simulink model "aero_pendulum_state_space"  (R2014a)
settings: Solver=ode45  StartTime=0.0  StopTime=Tsym  MaxStep=Ts  RelTol=1e-3
values from neighbouring files (symbols this model uses):
  A = [0 1; -m*l*g*d/J -c/J]    [paramters.m]
  B = [0; Km/J]    [paramters.m]
  C = [1 0]    [paramters.m]
  teta = 90    [paramters.m]
libraries: simulink x1
settings Model: Creator=Barti  LastModifiedBy=Barti

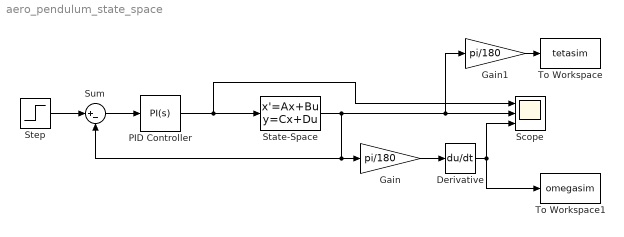
== system aero_pendulum_state_space ==
  Derivative : Derivative
  Gain : Gain  Gain=pi/180
  Gain1 : Gain  Gain=pi/180
  PID Controller : simulink/Continuous/PID Controller  Controller=PI  TimeDomain=Continuous-time  SampleTime=1  IntegratorMethod=Forward Euler  FilterMethod=Forward Euler  Form=Parallel  P=0.0280664414027214  I=0.0228225324869861  D=0  N=100  InitialConditionSource=internal  InitialConditionForIntegrator=0  InitialConditionForFilter=0  ExternalReset=none  LimitOutput=off  UpperSaturationLimit=inf  LowerSaturationLimit=-inf  LinearizeAsGain=on  AntiWindupMode=none  Kb=1  TrackingMode=off  Kt=1  PParamMin=[]  PParamMax=[]  IParamMin=[]  IParamMax=[]  DParamMin=[]  DParamMax=[]  NParamMin=[]  NParamMax=[]  KbParamMin=[]  KbParamMax=[]  KtParamMin=[]  KtParamMax=[]  POutMin=[]  POutMax=[]  IOutMin=[]  IOutMax=[]  DOutMin=[]  DOutMax=[]  NOutMin=[]  NOutMax=[]  KbOutMin=[]  KbOutMax=[]  KtOutMin=[]  KtOutMax=[]  IntegratorOutMin=[]  IntegratorOutMax=[]  FilterOutMin=[]  FilterOutMax=[]  SumOutMin=[]  SumOutMax=[]  SumI1OutMin=[]  SumI1OutMax=[]  SumI2OutMin=[]  SumI2OutMax=[]  SumI3OutMin=[]  SumI3OutMax=[]  SumDOutMin=[]  SumDOutMax=[]  SaturationOutMin=[]  SaturationOutMax=[]  IntegratorContinuousStateAttributes=''  IntegratorStateMustResolveToSignalObject=off  IntegratorRTWStateStorageClass=Auto  FilterContinuousStateAttributes=''  FilterStateMustResolveToSignalObject=off  FilterRTWStateStorageClass=Auto
  Scope : Scope  NumInputPorts=3
      settings: TimeRange=60  YMin=0~0~-5  YMax=3.5~16~5
  State-Space : StateSpace  A=A  B=B  C=C  D=0  X0=0
  Step : Step  Time=0  After=teta  SampleTime=0
  Sum : Sum  Inputs=|+-
  To Workspace : ToWorkspace  VariableName=tetasim  SampleTime=-1
  To Workspace1 : ToWorkspace  VariableName=omegasim  SampleTime=-1
  wires:
  PID Controller/1 -> Scope/1, State-Space/1
  State-Space/1 -> Gain1/1, Scope/2, Gain/1, Sum/2
  Sum/1 -> PID Controller/1
  Step/1 -> Sum/1
  Derivative/1 -> Scope/3, To Workspace1/1
  Gain/1 -> Derivative/1
  Gain1/1 -> To Workspace/1
